simulink model "MPCisnm"  (R2023a)
settings: Solver=ode4  StartTime=0.0  StopTime=tsim  FixedStep=baseRate  RelTol=1e-6  AbsTol=1e-6
values from neighbouring files (symbols this model uses):
  ALGORITHM = 6    [Run_Initializer.m]
  con0 = [n*N, 2*N, N, N, N]    [Run_Initializer.m]
  Gamma1_el = 0.12    [Run_Initializer.m]
  Gamma1_sh = 0.005    [Run_Initializer.m]
  Gamma1_wr = 0.025    [Run_Initializer.m]
  Gamma2_el = 5    [Run_Initializer.m]
  Gamma2_sh = 5    [Run_Initializer.m]
  Gamma2_wr = 5    [Run_Initializer.m]
  Gamma3_el = 10    [Run_Initializer.m]
  Gamma3_sh = 40    [Run_Initializer.m]
  Gamma3_wr = 40    [Run_Initializer.m]
  Gamma4_el = 0.039    [Run_Initializer.m]
  Gamma4_sh = 0.015    [Run_Initializer.m]
  Gamma4_wr = 0.029    [Run_Initializer.m]
  Gamma5_el = 800    [Run_Initializer.m]
  Gamma5_sh = 800    [Run_Initializer.m]
  Gamma5_wr = 800    [Run_Initializer.m]
  Gamma6_el = 0.000001    (= 1e-06)    [Run_Initializer.m]
  Gamma6_sh = 0.005    [Run_Initializer.m]
  Gamma6_wr = 0.02    [Run_Initializer.m]
  init_states_BLACK = [ct;thetat0].'    [Run_Initializer.m]
  init_states_BLUE = [pobj1;0].'    [Run_Initializer.m]
  init_states_RED = xi(1:3).'    [Run_Initializer.m]
  Kd_elarm = 0.8    [Run_Initializer.m]
  Kd_sharm = 1.0    (= 1)    [Run_Initializer.m]
  Kd_wrarm = 0.6    [Run_Initializer.m]
  Kp_elarm = 1.2    [Run_Initializer.m]
  Kp_sharm = 1.5    [Run_Initializer.m]
  Kp_wrarm = 2    [Run_Initializer.m]
  maxiterations = 10    [Run_Initializer.m]
  N = 15    [Run_Initializer.m]    (also in theFastMPCSolver2.m = length(z)/9)
  Phi = 2*H + kappa*P.'*d2*P    [theFastMPCSolver2.m]
  Td = 2    [Run_Initializer.m]
  thetat_dot = 2.5 * d2r    (= 0.0436332312999)    [Run_Initializer.m]
  tol = 0.00015    [Run_Initializer.m]
  Tz_lim_elarm = .1    (= 0.1)    [Run_Initializer.m]
  Tz_lim_sharm = .1    (= 0.1)    [Run_Initializer.m]
  Tz_lim_wrarm = .1    (= 0.1)    [Run_Initializer.m]
  vobj1 = [0.00;0.00]    [Run_Initializer.m]
  vtar = [-0.005;0.005]    [Run_Initializer.m]
undefined symbols (not defined in the file or in its folder): a1, a2, a3, Ad, b0, b1, b2, b3, baseRate, cdockdeltax, cdockoa, Cmat, DiscIntNeverNeededParam, drop_states_ARM, drop_states_BLACK, drop_states_BLUE, drop_states_RED, ecoa, F_Black_X_nominal, F_Black_Y_nominal, F_Blue_X_nominal, F_Blue_Y_nominal, F_red_X_nominal, F_red_Y_nominal, F_thrusters_BLACK, F_thrusters_BLUE, F_thrusters_RED, Fmat, gamma, H, IBLACK, IBLUE, IDIST, IEE, IPROX, IRED, Kd_tb, Kd_tblue, Kd_tr, Kd_xb, Kd_xblue, Kd_xr, Kd_yb, Kd_yblue, Kd_yr, KOZ_actual, Kp_tb, Kp_tblue, Kp_tr, Kp_xb, Kp_xblue, Kp_xr, Kp_yb, Kp_yblue, Kp_yr, mBLACK, mBLUE, mDIST, mEE, mPROX ... (+31)
libraries: nvidiaSharedBlocks x8, simulink x8, dspsigops x6, dspstat3 x5, MainLibrary x4
(part 3 of 10)

== system MPCisnm/Phase #3: Experiment/Change BLUE Behavior ==
  Action Port : ActionPort  ActionPortLabel=if(u1 == 3 | u2 == 1)
  Constant1 : Constant  Value=Phase3_SubPhase2_End  SampleTime=-1
  Constant2 : Constant  Value=Phase3_SubPhase3_End  SampleTime=-1
  Constant3 : Constant  Value=Phase3_SubPhase4_End  SampleTime=-1
  Constant4 : Constant  Value=Phase3_SubPhase1_End  SampleTime=-1
  Experiment Sub-Phases : If  NumInputs=5  IfExpression=u1 < u2  ElseIfExpressions=(u1 < u3 & u1 >= u2),(u1 < u4 & u1 >= u3), (u1 < u5 & u1 >= u4)  ShowElse=off
  Sub-Phase #1 : Subsystem  TreatAsAtomicUnit=on
  "Sub-Phase #2 " : Subsystem  TreatAsAtomicUnit=on
  "Sub-Phase #3 " : Subsystem  TreatAsAtomicUnit=on
  Sub-Phase #4 : Subsystem  TreatAsAtomicUnit=on
  Universal_Time : DataStoreRead  DataStoreName=Univ_Time  IndexOptions=Index vector (dialog)  Indices=1  OutputSizes=1
  wires:
  Constant3/1 -> Experiment Sub-Phases/5
  Experiment Sub-Phases/4 -> Sub-Phase #4/Action
  Universal_Time/1 -> Experiment Sub-Phases/1
  Experiment Sub-Phases/1 -> Sub-Phase #1/Action
  Constant2/1 -> Experiment Sub-Phases/4
  Constant4/1 -> Experiment Sub-Phases/2
  Constant1/1 -> Experiment Sub-Phases/3
  Experiment Sub-Phases/3 -> "Sub-Phase #3 "/Action
  Experiment Sub-Phases/2 -> "Sub-Phase #2 "/Action

== system MPCisnm/Phase #3: Experiment/Change RED Behavior ==
  note: For experiments, it is usually desirable to have various sub-phases. The sub-phases are defined in the initializer; note that in the template only three sub-phases are present, but more can be added.
  Action Port : ActionPort  ActionPortLabel=if(u1 == 1 | u2 == 1)
  Constant1 : Constant  Value=Phase3_SubPhase2_End  SampleTime=-1
  Constant2 : Constant  Value=Phase3_SubPhase3_End  SampleTime=-1
  Constant3 : Constant  Value=Phase3_SubPhase4_End  SampleTime=-1
  Constant4 : Constant  Value=Phase3_SubPhase1_End  SampleTime=-1
  Experiment Sub-Phases : If  NumInputs=5  IfExpression=u1 < u2  ElseIfExpressions=(u1 < u3 & u1 >= u2),(u1 < u4 & u1 >= u3), (u1 < u5 & u1 >= u4)  ShowElse=off
  Sub-Phase #1 : Subsystem  TreatAsAtomicUnit=on
  "Sub-Phase #2 " : Subsystem  TreatAsAtomicUnit=on
  "Sub-Phase #3 " : Subsystem  TreatAsAtomicUnit=on
  Sub-Phase #4 : Subsystem  TreatAsAtomicUnit=on
  Universal_Time : DataStoreRead  DataStoreName=Univ_Time  IndexOptions=Index vector (dialog)  Indices=1  OutputSizes=1
  wires:
  Experiment Sub-Phases/1 -> Sub-Phase #1/Action
  Experiment Sub-Phases/2 -> "Sub-Phase #2 "/Action
  Universal_Time/1 -> Experiment Sub-Phases/1
  Experiment Sub-Phases/3 -> "Sub-Phase #3 "/Action
  Constant4/1 -> Experiment Sub-Phases/2
  Constant1/1 -> Experiment Sub-Phases/3
  Constant2/1 -> Experiment Sub-Phases/4
  Constant3/1 -> Experiment Sub-Phases/5
  Experiment Sub-Phases/4 -> Sub-Phase #4/Action

== system MPCisnm/Phase #4: Return Home/Change BLACK Behavior ==
  note: Additional Blocks
  note: PD Control Law - BLACK
  note: Additional blocks are stored here.
  note: A simple PD control law is used here to command the platform to it's initial position, as defined in the initializer.
  Action Port : ActionPort  ActionPortLabel=if(u1 == 2 | u2 == 1)
  BLACK_Fx : DataStoreWrite  DataStoreName=BLACK_Fx  IndexOptions=Index vector (dialog)  Indices=1  OutputSizes=1
  BLACK_Fy : DataStoreWrite  DataStoreName=BLACK_Fy  IndexOptions=Index vector (dialog)  Indices=1  OutputSizes=1
  BLACK_Tz : DataStoreWrite  DataStoreName=BLACK_Tz  IndexOptions=Index vector (dialog)  Indices=1  OutputSizes=1
  Constant : Constant  Value=0
  Data Store Write3 : DataStoreWrite  DataStoreName=Float_State  IndexOptions=Index vector (dialog)  Indices=1  OutputSizes=1
  Puck State : Constant
  wires:
  Puck State/1 -> Data Store Write3/1
  Constant/1 -> BLACK_Fx/1, BLACK_Fy/1, BLACK_Tz/1

== system MPCisnm/Phase #4: Return Home/Change BLUE Behavior ==
  note: PD Control Law - BLUE
  note: Additional blocks are stored here.
  note: A simple PD control law is used here to command the platform to it's initial position, as defined in the initializer.
  note: Additional Blocks
  Action Port : ActionPort  ActionPortLabel=if(u1 == 3 | u2 == 1)
  BLUE_Fx : DataStoreWrite  DataStoreName=BLUE_Fx  IndexOptions=Index vector (dialog)  Indices=1  OutputSizes=1
  BLUE_Fy : DataStoreWrite  DataStoreName=BLUE_Fy  IndexOptions=Index vector (dialog)  Indices=1  OutputSizes=1
  BLUE_Tz : DataStoreWrite  DataStoreName=BLUE_Tz  IndexOptions=Index vector (dialog)  Indices=1  OutputSizes=1
  Constant : Constant  Value=0
  Data Store Write3 : DataStoreWrite  DataStoreName=Float_State  IndexOptions=Index vector (dialog)  Indices=1  OutputSizes=1
  Puck State : Constant
  wires:
  Puck State/1 -> Data Store Write3/1
  Constant/1 -> BLUE_Tz/1, BLUE_Fx/1, BLUE_Fy/1

== system MPCisnm/Phase #4: Return Home/Change RED Behavior ==
  note: PD Control Law - RED
  note: Additional Blocks
  note: Additional blocks are stored above. Note that to control attitude using the RW, simply replace RED_Tz with RED_Tz_RW.
  note: A simple PD control law is used here to command the platform to it's initial position, as defined in the initializer.
  note: ARM Control Law - RED
  Action Port : ActionPort  ActionPortLabel=if(u1 == 1 | u2 == 1)
  Constant{,1..3,5..7} (7 alike) : Constant  Value=0
  Constant4 : Constant  Commented=on  Value=platformSelection
  Data Store Write : DataStoreWrite  DataStoreName=MPC_State  IndexOptions=Index vector (dialog)  Indices=1  OutputSizes=1
  Data Store Write1 : DataStoreWrite  DataStoreName=RED_ARM_Control_Mode  IndexOptions=Index vector (dialog)  Indices=1  OutputSizes=1
  Data Store Write3 : DataStoreWrite  DataStoreName=Float_State  IndexOptions=Index vector (dialog)  Indices=1  OutputSizes=1
  If : If  Commented=on  IfExpression=u1 == 4 | u1 == 5 | u1 == 10 | u1 == 11  ShowElse=off
  Puck State : Constant
  RED+ARM : Subsystem  Commented=on  TreatAsAtomicUnit=on
  RED_Fx : DataStoreWrite  DataStoreName=RED_Fx  IndexOptions=Index vector (dialog)  Indices=1  OutputSizes=1
  RED_Fy : DataStoreWrite  DataStoreName=RED_Fy  IndexOptions=Index vector (dialog)  Indices=1  OutputSizes=1
  RED_Tz : DataStoreWrite  DataStoreName=RED_Tz  IndexOptions=Index vector (dialog)  Indices=1  OutputSizes=1
  RED_Tz_RW : DataStoreWrite  DataStoreName=RED_Tz_RW  IndexOptions=Index vector (dialog)  Indices=1  OutputSizes=1
  RED_Tz_RW1 : DataStoreWrite  DataStoreName=RED_Tz_RW  IndexOptions=Index vector (dialog)  Indices=1  OutputSizes=1
  wires:
  Constant2/1 -> RED_Tz_RW1/1
  Puck State/1 -> Data Store Write3/1
  Constant4/1 -> If/1
  If/1 -> RED+ARM/Action
  Constant1/1 -> RED_Fy/1
  Constant/1 -> RED_Fx/1
  Constant3/1 -> RED_Tz/1
  Constant5/1 -> RED_Tz_RW/1
  Constant6/1 -> Data Store Write1/1
  Constant7/1 -> Data Store Write/1

== system MPCisnm/Phase #5: Hold Home/Change BLACK Behavior ==
  note: Additional Blocks
  note: PD Control Law - BLACK
  note: Additional blocks are stored here.
  note: A simple PD control law is used here to command the platform to it's initial position, as defined in the initializer.
  Action Port : ActionPort  ActionPortLabel=if(u1 == 2 | u2 == 1)
  BLACK_Fx : DataStoreWrite  DataStoreName=BLACK_Fx  IndexOptions=Index vector (dialog)  Indices=1  OutputSizes=1
  BLACK_Fy : DataStoreWrite  DataStoreName=BLACK_Fy  IndexOptions=Index vector (dialog)  Indices=1  OutputSizes=1
  BLACK_Tz : DataStoreWrite  DataStoreName=BLACK_Tz  IndexOptions=Index vector (dialog)  Indices=1  OutputSizes=1
  Data Store Write3 : DataStoreWrite  DataStoreName=Float_State  IndexOptions=Index vector (dialog)  Indices=1  OutputSizes=1
  Puck State : Constant
  Puck State1 : Constant  Value=0
  Puck State2 : Constant  Value=0
  Puck State3 : Constant  Value=0
  wires:
  Puck State2/1 -> BLACK_Fy/1
  Puck State3/1 -> BLACK_Tz/1
  Puck State1/1 -> BLACK_Fx/1
  Puck State/1 -> Data Store Write3/1

== system MPCisnm/Phase #5: Hold Home/Change BLUE Behavior ==
  note: PD Control Law - BLUE
  note: Additional blocks are stored here.
  note: A simple PD control law is used here to command the platform to it's initial position, as defined in the initializer.
  note: Additional Blocks
  Action Port : ActionPort  ActionPortLabel=if(u1 == 3 | u2 == 1)
  BLUE_Fx : DataStoreWrite  DataStoreName=BLUE_Fx  IndexOptions=Index vector (dialog)  Indices=1  OutputSizes=1
  BLUE_Fy : DataStoreWrite  DataStoreName=BLUE_Fy  IndexOptions=Index vector (dialog)  Indices=1  OutputSizes=1
  BLUE_Tz : DataStoreWrite  DataStoreName=BLUE_Tz  IndexOptions=Index vector (dialog)  Indices=1  OutputSizes=1
  Data Store Write3 : DataStoreWrite  DataStoreName=Float_State  IndexOptions=Index vector (dialog)  Indices=1  OutputSizes=1
  Puck State : Constant
  Puck State1 : Constant  Value=0
  Puck State2 : Constant  Value=0
  Puck State3 : Constant  Value=0
  wires:
  Puck State/1 -> Data Store Write3/1
  Puck State1/1 -> BLUE_Fx/1
  Puck State3/1 -> BLUE_Tz/1
  Puck State2/1 -> BLUE_Fy/1

== system MPCisnm/Phase #5: Hold Home/Change RED Behavior ==
  note: PD Control Law - RED
  note: Additional Blocks
  note: Additional blocks are stored above. Note that to control attitude using the RW, simply replace RED_Tz with RED_Tz_RW.
  note: A simple PD control law is used here to command the platform to it's initial position, as defined in the initializer.
  note: ARM Control Law - RED
  Action Port : ActionPort  ActionPortLabel=if(u1 == 1 | u2 == 1)
  Constant{,1..3,5..7} (7 alike) : Constant  Value=0
  Constant4 : Constant  Commented=on  Value=platformSelection
  Data Store Write : DataStoreWrite  DataStoreName=MPC_State  IndexOptions=Index vector (dialog)  Indices=1  OutputSizes=1
  Data Store Write1 : DataStoreWrite  DataStoreName=RED_ARM_Control_Mode  IndexOptions=Index vector (dialog)  Indices=1  OutputSizes=1
  Data Store Write3 : DataStoreWrite  DataStoreName=Float_State  IndexOptions=Index vector (dialog)  Indices=1  OutputSizes=1
  If : If  Commented=on  IfExpression=u1 == 4 | u1 == 5 | u1 == 10 | u1 == 11  ShowElse=off
  Puck State : Constant
  RED+ARM : Subsystem  Commented=on  TreatAsAtomicUnit=on
  RED_Fx : DataStoreWrite  DataStoreName=RED_Fx  IndexOptions=Index vector (dialog)  Indices=1  OutputSizes=1
  RED_Fy : DataStoreWrite  DataStoreName=RED_Fy  IndexOptions=Index vector (dialog)  Indices=1  OutputSizes=1
  RED_Tz : DataStoreWrite  DataStoreName=RED_Tz  IndexOptions=Index vector (dialog)  Indices=1  OutputSizes=1
  RED_Tz_RW : DataStoreWrite  DataStoreName=RED_Tz_RW  IndexOptions=Index vector (dialog)  Indices=1  OutputSizes=1
  RED_Tz_RW1 : DataStoreWrite  DataStoreName=RED_Tz_RW  IndexOptions=Index vector (dialog)  Indices=1  OutputSizes=1
  wires:
  Constant2/1 -> RED_Tz_RW1/1
  Puck State/1 -> Data Store Write3/1
  Constant4/1 -> If/1
  If/1 -> RED+ARM/Action
  Constant1/1 -> RED_Fy/1
  Constant/1 -> RED_Fx/1
  Constant3/1 -> RED_Tz/1
  Constant5/1 -> RED_Tz_RW/1
  Constant6/1 -> Data Store Write1/1
  Constant7/1 -> Data Store Write/1

== system MPCisnm/Phase #6: Clean Shutdown/Change BLACK Behavior ==
  note: At the end of the experiment, the pucks must be turned off.
  note: At the end of the experiment, all thrust and arms movement must cease.
  Action Port : ActionPort  ActionPortLabel=if(u1 == 2 | u2 == 1)
  BLACK_Fx : DataStoreWrite  DataStoreName=BLACK_Fx  IndexOptions=Index vector (dialog)  Indices=1  OutputSizes=1
  BLACK_Fy : DataStoreWrite  DataStoreName=BLACK_Fy  IndexOptions=Index vector (dialog)  Indices=1  OutputSizes=1
  BLACK_Tz : DataStoreWrite  DataStoreName=BLACK_Tz  IndexOptions=Index vector (dialog)  Indices=1  OutputSizes=1
  Constant3 : Constant  Value=0
  Constant4 : Constant  Value=0
  Constant5 : Constant  Value=0
  Data Store Write3 : DataStoreWrite  DataStoreName=Float_State  IndexOptions=Index vector (dialog)  Indices=1  OutputSizes=1
  Puck State : Constant  Value=0
  wires:
  Constant3/1 -> BLACK_Fx/1
  Constant5/1 -> BLACK_Tz/1
  Constant4/1 -> BLACK_Fy/1
  Puck State/1 -> Data Store Write3/1

== system MPCisnm/Phase #6: Clean Shutdown/Change BLUE Behavior ==
  note: Before getting good data, the platforms must NOT be floating. So, float is set to be "off".
  note: For the initialization phase, we do not want any thrust. Thus, all commanded forces are zero.
  Action Port : ActionPort  ActionPortLabel=if(u1 == 3 | u2 == 1)
  BLUE_Fx : DataStoreWrite  DataStoreName=BLUE_Fx  IndexOptions=Index vector (dialog)  Indices=1  OutputSizes=1
  BLUE_Fy : DataStoreWrite  DataStoreName=BLUE_Fy  IndexOptions=Index vector (dialog)  Indices=1  OutputSizes=1
  BLUE_Tz : DataStoreWrite  DataStoreName=BLUE_Tz  IndexOptions=Index vector (dialog)  Indices=1  OutputSizes=1
  Constant3 : Constant  Value=0
  Constant4 : Constant  Value=0
  Constant5 : Constant  Value=0
  Data Store Write4 : DataStoreWrite  DataStoreName=Float_State  IndexOptions=Index vector (dialog)  Indices=1  OutputSizes=1
  Puck State : Constant  Value=0
  wires:
  Constant3/1 -> BLUE_Fx/1
  Constant5/1 -> BLUE_Tz/1
  Constant4/1 -> BLUE_Fy/1
  Puck State/1 -> Data Store Write4/1

== system MPCisnm/Phase #6: Clean Shutdown/Change RED Behavior ==
  note: At the end of the experiment, the pucks must be turned off.
  note: At the end of the experiment, all thrust and arms movement must cease.
  note: Once the platform has settled, the RW must be slowly desaturated (assuming it has been used).
  Action Port : ActionPort  ActionPortLabel=if(u1 == 1 | u2 == 1)
  Constant{,1..3,7} (5 alike) : Constant  Value=0
  Data Store Write : DataStoreWrite  DataStoreName=MPC_State  IndexOptions=Index vector (dialog)  Indices=1  OutputSizes=1
  Data Store Write1 : DataStoreWrite  DataStoreName=RED_ARM_Control_Mode  IndexOptions=Index vector (dialog)  Indices=1  OutputSizes=1
  Data Store Write3 : DataStoreWrite  DataStoreName=Float_State  IndexOptions=Index vector (dialog)  Indices=1  OutputSizes=1
  Gain : Gain  Gain=-1
  Puck State : Constant  Value=0
  RED_Fx : DataStoreWrite  DataStoreName=RED_Fx  IndexOptions=Index vector (dialog)  Indices=1  OutputSizes=1
  RED_Fy : DataStoreWrite  DataStoreName=RED_Fy  IndexOptions=Index vector (dialog)  Indices=1  OutputSizes=1
  RED_Tz : DataStoreWrite  DataStoreName=RED_Tz  IndexOptions=Index vector (dialog)  Indices=1  OutputSizes=1
  RED_Tz_RW : DataStoreWrite  DataStoreName=RED_Tz_RW  IndexOptions=Index vector (dialog)  Indices=1  OutputSizes=1
  RED_dRz_Speed : DataStoreRead  DataStoreName=RED_dRz_RW_Sat  IndexOptions=Index vector (dialog)  Indices=1  OutputSizes=1
  Saturation : Saturate  UpperLimit=0.005  LowerLimit=-0.005
  wires:
  Constant/1 -> RED_Fx/1
  RED_dRz_Speed/1 -> Gain/1
  Saturation/1 -> RED_Tz_RW/1
  Constant1/1 -> RED_Fy/1
  Gain/1 -> Saturation/1
  Constant2/1 -> RED_Tz/1
  Puck State/1 -> Data Store Write3/1
  Constant3/1 -> Data Store Write1/1
  Constant7/1 -> Data Store Write/1

== system MPCisnm/PhaseSpace Camera Code/Initialize Universal Time (Simulation) ==
  Action Port : ActionPort  ActionPortLabel=elseif(u1 == 1)
  Set Universal Time (If this is a simulation) : Clock
  Universal_Time : DataStoreWrite  DataStoreName=Univ_Time  IndexOptions=Index vector (dialog)  Indices=1  OutputSizes=1
  wires:
  Set Universal Time (If this is a simulation)/1 -> Universal_Time/1

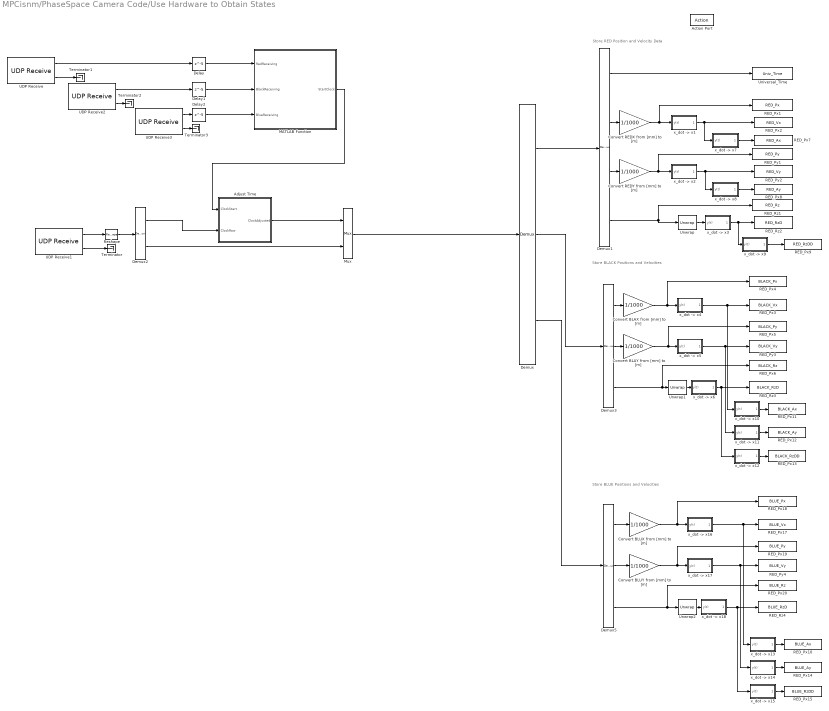
== system MPCisnm/PhaseSpace Camera Code/Use Hardware to Obtain States ==
  note: Store RED Position and Velocity Data
  note: Store BLUE Positions and Velocities
  note: Store BLACK Positions and Velocities
  Action Port : ActionPort  ActionPortLabel=if(u1 == 0)
  Adjust Time : Subsystem
  Convert BLAX from [mm] to [m] : Gain  Gain=1/1000
  Convert BLAY from [mm] to [m] : Gain  Gain=1/1000
  Convert BLUX from [mm] to [m] : Gain  Gain=1/1000
  Convert BLUY from [mm] to [m] : Gain  Gain=1/1000
  Convert REDX from [mm] to [m] : Gain  Gain=1/1000
  Convert REDY from [mm] to [m] : Gain  Gain=1/1000
  Delay : Delay  DelayLength=5
  Delay1 : Delay  DelayLength=5
  Delay2 : Delay  DelayLength=5
  Demux : Demux  Outputs=[4,3,3]
  Demux1 : Demux
  Demux2 : Demux  Outputs=[1,9]
  Demux3 : Demux  Outputs=3
  Demux5 : Demux  Outputs=3
  MATLAB Function : MATLAB Function  TreatAsAtomicUnit=on
  Mux : Mux  Inputs=2
  RED_Px1 : DataStoreWrite  DataStoreName=RED_Px  IndexOptions=Index vector (dialog)  Indices=1  OutputSizes=1
  RED_Px10 : DataStoreWrite  DataStoreName=BLUE_Ax  IndexOptions=Index vector (dialog)  Indices=1  OutputSizes=1
  RED_Px11 : DataStoreWrite  DataStoreName=BLACK_Ax  IndexOptions=Index vector (dialog)  Indices=1  OutputSizes=1
  RED_Px12 : DataStoreWrite  DataStoreName=BLACK_Ay  IndexOptions=Index vector (dialog)  Indices=1  OutputSizes=1
  RED_Px13 : DataStoreWrite  DataStoreName=BLACK_RzDD  IndexOptions=Index vector (dialog)  Indices=1  OutputSizes=1
  RED_Px14 : DataStoreWrite  DataStoreName=BLUE_Ay  IndexOptions=Index vector (dialog)  Indices=1  OutputSizes=1
  RED_Px15 : DataStoreWrite  DataStoreName=BLUE_RzDD  IndexOptions=Index vector (dialog)  Indices=1  OutputSizes=1
  RED_Px17 : DataStoreWrite  DataStoreName=BLUE_Vx  IndexOptions=Index vector (dialog)  Indices=1  OutputSizes=1
  RED_Px18 : DataStoreWrite  DataStoreName=BLUE_Px  IndexOptions=Index vector (dialog)  Indices=1  OutputSizes=1
  RED_Px19 : DataStoreWrite  DataStoreName=BLUE_Py  IndexOptions=Index vector (dialog)  Indices=1  OutputSizes=1
  RED_Px2 : DataStoreWrite  DataStoreName=RED_Vx  IndexOptions=Index vector (dialog)  Indices=1  OutputSizes=1
  RED_Px20 : DataStoreWrite  DataStoreName=BLUE_Rz  IndexOptions=Index vector (dialog)  Indices=1  OutputSizes=1
  RED_Px3 : DataStoreWrite  DataStoreName=BLACK_Vx  IndexOptions=Index vector (dialog)  Indices=1  OutputSizes=1
  RED_Px4 : DataStoreWrite  DataStoreName=BLACK_Px  IndexOptions=Index vector (dialog)  Indices=1  OutputSizes=1
  RED_Px5 : DataStoreWrite  DataStoreName=BLACK_Py  IndexOptions=Index vector (dialog)  Indices=1  OutputSizes=1
  RED_Px6 : DataStoreWrite  DataStoreName=BLACK_Rz  IndexOptions=Index vector (dialog)  Indices=1  OutputSizes=1
  RED_Px7 : DataStoreWrite  DataStoreName=RED_Ax  IndexOptions=Index vector (dialog)  Indices=1  OutputSizes=1
  RED_Px8 : DataStoreWrite  DataStoreName=RED_Ay  IndexOptions=Index vector (dialog)  Indices=1  OutputSizes=1
  RED_Px9 : DataStoreWrite  DataStoreName=RED_RzDD  IndexOptions=Index vector (dialog)  Indices=1  OutputSizes=1
  RED_Py1 : DataStoreWrite  DataStoreName=RED_Py  IndexOptions=Index vector (dialog)  Indices=1  OutputSizes=1
  RED_Py2 : DataStoreWrite  DataStoreName=RED_Vy  IndexOptions=Index vector (dialog)  Indices=1  OutputSizes=1
  RED_Py3 : DataStoreWrite  DataStoreName=BLACK_Vy  IndexOptions=Index vector (dialog)  Indices=1  OutputSizes=1
  RED_Py4 : DataStoreWrite  DataStoreName=BLUE_Vy  IndexOptions=Index vector (dialog)  Indices=1  OutputSizes=1
  RED_Rz1 : DataStoreWrite  DataStoreName=RED_Rz  IndexOptions=Index vector (dialog)  Indices=1  OutputSizes=1
  RED_Rz2 : DataStoreWrite  DataStoreName=RED_RzD  IndexOptions=Index vector (dialog)  Indices=1  OutputSizes=1
  RED_Rz3 : DataStoreWrite  DataStoreName=BLACK_RzD  IndexOptions=Index vector (dialog)  Indices=1  OutputSizes=1
  RED_Rz4 : DataStoreWrite  DataStoreName=BLUE_RzD  IndexOptions=Index vector (dialog)  Indices=1  OutputSizes=1
  Reshape : Reshape  OutputDimensionality=Customize  OutputDimensions=[10,1]
  Terminator{,1..3} (4 alike) : Terminator
  UDP Receive : nvidiaSharedBlocks/UDP Receive  localURL='0.0.0.0'  localPort=33001  remoteURL='0.0.0.0'  remotePort=-1  recvBufferSize=8192  signalDatatype=int32  dims=1  isVarSize=off  showBlockingTime=off  blockingTime=0  sampletime=-1  blockPlatform=NVIDIA
      settings: LibrarySourceBlock=nvidiaNetworklib/UDP Receive
  UDP Receive1 : nvidiaSharedBlocks/UDP Receive  localURL='0.0.0.0'  localPort=31534  remoteURL='0.0.0.0'  remotePort=-1  recvBufferSize=8192  signalDatatype=double  dims=10  isVarSize=off  showBlockingTime=off  blockingTime=0  sampletime=-1  blockPlatform=NVIDIA
  UDP Receive2 : nvidiaSharedBlocks/UDP Receive  localURL='0.0.0.0'  localPort=33002  remoteURL='0.0.0.0'  remotePort=-1  recvBufferSize=8192  signalDatatype=int32  dims=1  isVarSize=off  showBlockingTime=off  blockingTime=0  sampletime=-1  blockPlatform=NVIDIA
      settings: LibrarySourceBlock=nvidiaNetworklib/UDP Receive
  UDP Receive3 : nvidiaSharedBlocks/UDP Receive  localURL='0.0.0.0'  localPort=33003  remoteURL='0.0.0.0'  remotePort=-1  recvBufferSize=8192  signalDatatype=int32  dims=1  isVarSize=off  showBlockingTime=off  blockingTime=0  sampletime=-1  blockPlatform=NVIDIA
      settings: LibrarySourceBlock=nvidiaNetworklib/UDP Receive
  Universal_Time : DataStoreWrite  DataStoreName=Univ_Time  IndexOptions=Index vector (dialog)  Indices=1  OutputSizes=1
  Unwrap : dspsigops/Unwrap  tol=pi  InputProcessing=Columns as channels (frame based)  running=off
  Unwrap1 : dspsigops/Unwrap  tol=pi  InputProcessing=Columns as channels (frame based)  running=off
  Unwrap2 : dspsigops/Unwrap  tol=pi  InputProcessing=Columns as channels (frame based)  running=off
  "x_dot -> x1" : Subsystem
  "x_dot -> x10" : Subsystem
  "x_dot -> x11" : Subsystem
  "x_dot -> x12" : Subsystem
  "x_dot -> x13" : Subsystem
  "x_dot -> x14" : Subsystem
  "x_dot -> x15" : Subsystem
  "x_dot -> x16" : Subsystem
  "x_dot -> x17" : Subsystem
  "x_dot -> x18" : Subsystem
  "x_dot -> x2" : Subsystem
  "x_dot -> x3" : Subsystem
  "x_dot -> x4" : Subsystem
  "x_dot -> x5" : Subsystem
  "x_dot -> x6" : Subsystem
  "x_dot -> x7" : Subsystem
  "x_dot -> x8" : Subsystem
  "x_dot -> x9" : Subsystem
  wires:
  "x_dot -> x12"/1(dy(t)/dt) -> RED_Px13/1
  "x_dot -> x6"/1(dy(t)/dt) -> RED_Rz3/1, "x_dot -> x12"/1(y(t))
  Unwrap2/1 -> "x_dot -> x18"/1(y(t))
  Demux1/4 -> Unwrap/1, RED_Rz1/1
  Demux3/3 -> Unwrap1/1, RED_Px6/1
  Demux3/2 -> Convert BLAY from [mm] to [m]/1
  Demux5/2 -> Convert BLUY from [mm] to [m]/1
  "x_dot -> x1"/1(dy(t)/dt) -> "x_dot -> x7"/1(y(t)), RED_Px2/1
  Demux5/3 -> Unwrap2/1, RED_Px20/1
  Demux5/1 -> Convert BLUX from [mm] to [m]/1
  "x_dot -> x2"/1(dy(t)/dt) -> "x_dot -> x8"/1(y(t)), RED_Py2/1
  Demux1/3 -> Convert REDY from [mm] to [m]/1
  Demux/1 -> Demux1/1
  "x_dot -> x8"/1(dy(t)/dt) -> RED_Px8/1
  Unwrap/1 -> "x_dot -> x3"/1(y(t))
  Demux/2 -> Demux3/1
  "x_dot -> x10"/1(dy(t)/dt) -> RED_Px11/1
  "x_dot -> x3"/1(dy(t)/dt) -> "x_dot -> x9"/1(y(t)), RED_Rz2/1
  "x_dot -> x7"/1(dy(t)/dt) -> RED_Px7/1
  "x_dot -> x11"/1(dy(t)/dt) -> RED_Px12/1
  "x_dot -> x5"/1(dy(t)/dt) -> RED_Py3/1, "x_dot -> x11"/1(y(t))
  Unwrap1/1 -> "x_dot -> x6"/1(y(t))
  "x_dot -> x4"/1(dy(t)/dt) -> "x_dot -> x10"/1(y(t)), RED_Px3/1
  Demux3/1 -> Convert BLAX from [mm] to [m]/1
  Demux1/2 -> Convert REDX from [mm] to [m]/1
  "x_dot -> x9"/1(dy(t)/dt) -> RED_Px9/1
  UDP Receive1/1 -> Reshape/1
  UDP Receive1/2 -> Terminator/1
  Mux/1 -> Demux/1
  Demux/3 -> Demux5/1
  Convert REDX from [mm] to [m]/1 -> "x_dot -> x1"/1(y(t)), RED_Px1/1
  Convert REDY from [mm] to [m]/1 -> "x_dot -> x2"/1(y(t)), RED_Py1/1
  Convert BLAX from [mm] to [m]/1 -> "x_dot -> x4"/1(y(t)), RED_Px4/1
  Convert BLAY from [mm] to [m]/1 -> "x_dot -> x5"/1(y(t)), RED_Px5/1
  "x_dot -> x17"/1(dy(t)/dt) -> "x_dot -> x14"/1(y(t)), RED_Py4/1
  "x_dot -> x16"/1(dy(t)/dt) -> "x_dot -> x13"/1(y(t)), RED_Px17/1
  "x_dot -> x14"/1(dy(t)/dt) -> RED_Px14/1
  "x_dot -> x15"/1(dy(t)/dt) -> RED_Px15/1
  "x_dot -> x13"/1(dy(t)/dt) -> RED_Px10/1
  "x_dot -> x18"/1(dy(t)/dt) -> "x_dot -> x15"/1(y(t)), RED_Rz4/1
  Convert BLUX from [mm] to [m]/1 -> "x_dot -> x16"/1(y(t)), RED_Px18/1
  Convert BLUY from [mm] to [m]/1 -> "x_dot -> x17"/1(y(t)), RED_Px19/1
  Demux1/1 -> Universal_Time/1
  Reshape/1 -> Demux2/1
  Demux2/2 -> Mux/2
  Adjust Time/1(ClockAdjusted) -> Mux/1
  Demux2/1 -> Adjust Time/2(ClockRaw)
  UDP Receive3/2 -> Terminator3/1
  UDP Receive2/2 -> Terminator2/1
  UDP Receive/1 -> Delay/1
  UDP Receive/2 -> Terminator1/1
  UDP Receive3/1 -> Delay2/1
  UDP Receive2/1 -> Delay1/1
  Delay/1 -> MATLAB Function/1(RedReceiving)
  Delay1/1 -> MATLAB Function/2(BlackReceiving)
  Delay2/1 -> MATLAB Function/3(BlueReceiving)
  MATLAB Function/1(StartClock) -> Adjust Time/1(ClockStart)

== system MPCisnm/Platform Identification/Subsystem ==
  Action Port : ActionPort  ActionPortLabel=if(u1 == 0)
  Data Store Write : DataStoreWrite  DataStoreName=WhoAmI  IndexOptions=Index vector (dialog)  Indices=1  OutputSizes=1
  WhoAmI : MainLibrary/WhoAmI  SampleTime=baseRate
      settings: SourceProductName=SPOT Custom Library
  wires:
  WhoAmI/1 -> Data Store Write/1

== system MPCisnm/Robotic Arm Code/Change RED Behavior ==
  Action Port : ActionPort  ActionPortLabel=if(u1 == 1 & u2 == 0)
  Arm Control Mode : DataStoreRead  DataStoreName=RED_ARM_Control_Mode  IndexOptions=Index vector (dialog)  Indices=1  OutputSizes=1
  "Control Dynamixel Actuators in either Position, Current, or Speed Control Modes" : MainLibrary/Dynamixel Functions/Control Dynamixel Actuators in  either Position, Current, or Speed  Control Modes  POSITION_P_GAIN=400  POSITION_I_GAIN=0  POSITION_D_GAIN=200  MAX_POSITION=3072  MIN_POSITION=1024  MOVE_TIME=0  CURRENT_LIMIT=850  SPEED_P_GAIN=400  SPEED_I_GAIN=100  VELOCITY_LIMIT=50  ACCELERATION_TIME=0  SampleTime=baseRate
      settings: SourceProductName=SPOT Custom Library
  Elbow Command : DataStoreRead  DataStoreName=RED_Elbow_Command  IndexOptions=Index vector (dialog)  Indices=1  OutputSizes=1
  Shoulder Command : DataStoreRead  DataStoreName=RED_Shoulder_Command  IndexOptions=Index vector (dialog)  Indices=1  OutputSizes=1
  Wrist Command : DataStoreRead  DataStoreName=RED_Wrist_Command  IndexOptions=Index vector (dialog)  Indices=1  OutputSizes=1
  wires:
  Arm Control Mode/1 -> "Control Dynamixel Actuators in either Position, Current, or Speed Control Modes"/1
  Shoulder Command/1 -> "Control Dynamixel Actuators in either Position, Current, or Speed Control Modes"/2
  Elbow Command/1 -> "Control Dynamixel Actuators in either Position, Current, or Speed Control Modes"/3
  Wrist Command/1 -> "Control Dynamixel Actuators in either Position, Current, or Speed Control Modes"/4

== system MPCisnm/Send Data to TX2/Subsystem ==
  Action Port : ActionPort  ActionPortLabel=if(u1 == 0)
  BLACK_Px : DataStoreRead  DataStoreName=BLACK_Px  IndexOptions=Index vector (dialog)  Indices=1  OutputSizes=1
  BLACK_Py : DataStoreRead  DataStoreName=BLACK_Py  IndexOptions=Index vector (dialog)  Indices=1  OutputSizes=1
  BLACK_Rz : DataStoreRead  DataStoreName=BLACK_Rz  IndexOptions=Index vector (dialog)  Indices=1  OutputSizes=1
  BLACK_RzD : DataStoreRead  DataStoreName=BLACK_RzD  IndexOptions=Index vector (dialog)  Indices=1  OutputSizes=1
  BLACK_Vx : DataStoreRead  DataStoreName=BLACK_Vx  IndexOptions=Index vector (dialog)  Indices=1  OutputSizes=1
  BLACK_Vy : DataStoreRead  DataStoreName=BLACK_Vy  IndexOptions=Index vector (dialog)  Indices=1  OutputSizes=1
  BLUE_Px : DataStoreRead  DataStoreName=BLUE_Px  IndexOptions=Index vector (dialog)  Indices=1  OutputSizes=1
  BLUE_Py : DataStoreRead  DataStoreName=BLUE_Py  IndexOptions=Index vector (dialog)  Indices=1  OutputSizes=1
  BLUE_Rz : DataStoreRead  DataStoreName=BLUE_Rz  IndexOptions=Index vector (dialog)  Indices=1  OutputSizes=1
  BLUE_RzD : DataStoreRead  DataStoreName=BLUE_RzD  IndexOptions=Index vector (dialog)  Indices=1  OutputSizes=1
  BLUE_Vx : DataStoreRead  DataStoreName=BLUE_Vx  IndexOptions=Index vector (dialog)  Indices=1  OutputSizes=1
  BLUE_Vy : DataStoreRead  DataStoreName=BLUE_Vy  IndexOptions=Index vector (dialog)  Indices=1  OutputSizes=1
  Mux : Mux  Inputs=19
  RED_Px : DataStoreRead  DataStoreName=RED_Px  IndexOptions=Index vector (dialog)  Indices=1  OutputSizes=1
  "RED_Py " : DataStoreRead  DataStoreName=RED_Py  IndexOptions=Index vector (dialog)  Indices=1  OutputSizes=1
  RED_Rz : DataStoreRead  DataStoreName=RED_Rz  IndexOptions=Index vector (dialog)  Indices=1  OutputSizes=1
  "RED_Vx " : DataStoreRead  DataStoreName=RED_Vx  IndexOptions=Index vector (dialog)  Indices=1  OutputSizes=1
  RED_Vy : DataStoreRead  DataStoreName=RED_Vy  IndexOptions=Index vector (dialog)  Indices=1  OutputSizes=1
  RED_Vz : DataStoreRead  DataStoreName=RED_RzD  IndexOptions=Index vector (dialog)  Indices=1  OutputSizes=1
  Time : DataStoreRead  DataStoreName=Univ_Time  IndexOptions=Index vector (dialog)  Indices=1  OutputSizes=1
  UDP Send : nvidiaSharedBlocks/UDP Send  remoteURL='192.168.1.113'  remotePort=46875  localURL='0.0.0.0'  localPortSource=Automatically determine  localPort=-1  sampletime=-1  blockPlatform=NVIDIA  separateLengthPort=0
      settings: LibrarySourceBlock=nvidiaNetworklib/UDP Send
  wires:
  Mux/1 -> UDP Send/1
  BLUE_RzD/1 -> Mux/19
  Time/1 -> Mux/1
  RED_Px/1 -> Mux/2
  "RED_Py "/1 -> Mux/3
  RED_Rz/1 -> Mux/4
  "RED_Vx "/1 -> Mux/5
  RED_Vy/1 -> Mux/6
  RED_Vz/1 -> Mux/7
  BLACK_Px/1 -> Mux/8
  BLACK_Py/1 -> Mux/9
  BLACK_Rz/1 -> Mux/10
  BLACK_Vx/1 -> Mux/11
  BLACK_Vy/1 -> Mux/12
  BLACK_RzD/1 -> Mux/13
  BLUE_Px/1 -> Mux/14
  BLUE_Py/1 -> Mux/15
  BLUE_Rz/1 -> Mux/16
  BLUE_Vx/1 -> Mux/17
  BLUE_Vy/1 -> Mux/18

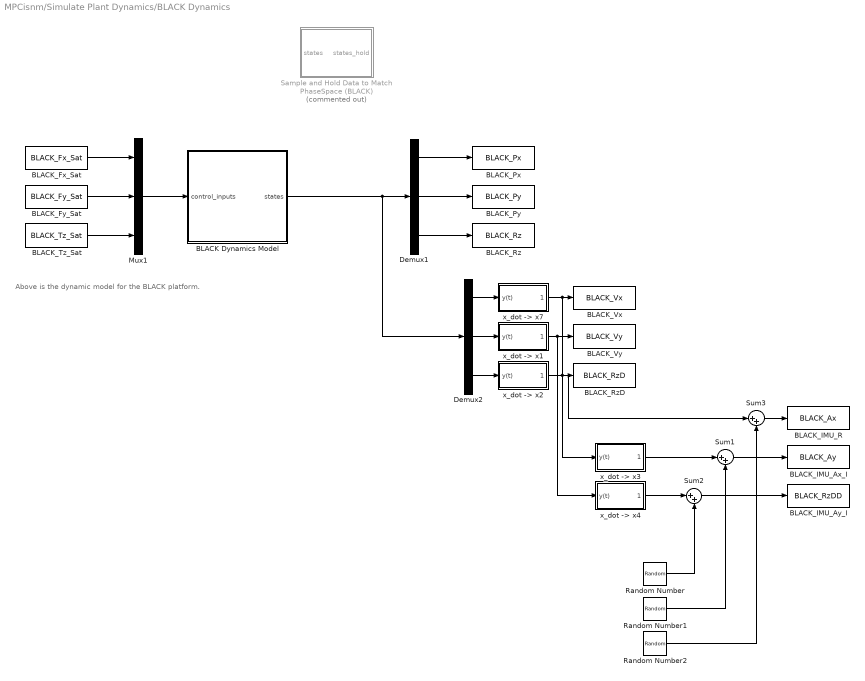
== system MPCisnm/Simulate Plant Dynamics/BLACK Dynamics ==
  note: Above is the dynamic model for the BLACK platform.
  BLACK Dynamics Model : Subsystem  SystemSampleTime=serverRate
  BLACK_Fx_Sat : DataStoreRead  DataStoreName=BLACK_Fx_Sat  IndexOptions=Index vector (dialog)  Indices=1  OutputSizes=1
  BLACK_Fy_Sat : DataStoreRead  DataStoreName=BLACK_Fy_Sat  IndexOptions=Index vector (dialog)  Indices=1  OutputSizes=1
  BLACK_IMU_Ax_I : DataStoreWrite  DataStoreName=BLACK_Ay  IndexOptions=Index vector (dialog)  Indices=1  OutputSizes=1
  BLACK_IMU_Ay_I : DataStoreWrite  DataStoreName=BLACK_RzDD  IndexOptions=Index vector (dialog)  Indices=1  OutputSizes=1
  BLACK_IMU_R : DataStoreWrite  DataStoreName=BLACK_Ax  IndexOptions=Index vector (dialog)  Indices=1  OutputSizes=1
  BLACK_Px : DataStoreWrite  DataStoreName=BLACK_Px  IndexOptions=Index vector (dialog)  Indices=1  OutputSizes=1
  BLACK_Py : DataStoreWrite  DataStoreName=BLACK_Py  IndexOptions=Index vector (dialog)  Indices=1  OutputSizes=1
  BLACK_Rz : DataStoreWrite  DataStoreName=BLACK_Rz  IndexOptions=Index vector (dialog)  Indices=1  OutputSizes=1
  BLACK_RzD : DataStoreWrite  DataStoreName=BLACK_RzD  IndexOptions=Index vector (dialog)  Indices=1  OutputSizes=1
  BLACK_Tz_Sat : DataStoreRead  DataStoreName=BLACK_Tz_Sat  IndexOptions=Index vector (dialog)  Indices=1  OutputSizes=1
  BLACK_Vx : DataStoreWrite  DataStoreName=BLACK_Vx  IndexOptions=Index vector (dialog)  Indices=1  OutputSizes=1
  BLACK_Vy : DataStoreWrite  DataStoreName=BLACK_Vy  IndexOptions=Index vector (dialog)  Indices=1  OutputSizes=1
  Demux1 : Demux  Outputs=3
  Demux2 : Demux  Outputs=3
  Mux1 : Mux  Inputs=3
  Random Number : RandomNumber  Variance=1.5e-6
  Random Number1 : RandomNumber  Variance=1.5e-6
  Random Number2 : RandomNumber  Variance=1.5e-6
  Sample and Hold Data to Match PhaseSpace (BLACK) : Subsystem  Commented=on
  Sum1 : Sum  Inputs=|++
  Sum2 : Sum  Inputs=|++
  Sum3 : Sum  Inputs=|++
  "x_dot -> x1" : Subsystem
  "x_dot -> x2" : Subsystem
  "x_dot -> x3" : Subsystem
  "x_dot -> x4" : Subsystem
  "x_dot -> x7" : Subsystem
  wires:
  BLACK_Fy_Sat/1 -> Mux1/2
  BLACK_Tz_Sat/1 -> Mux1/3
  Demux1/1 -> BLACK_Px/1
  "x_dot -> x7"/1(dy(t)/dt) -> "x_dot -> x3"/1(y(t)), BLACK_Vx/1
  "x_dot -> x2"/1(dy(t)/dt) -> Sum3/1, BLACK_RzD/1
  Demux1/2 -> BLACK_Py/1
  "x_dot -> x1"/1(dy(t)/dt) -> "x_dot -> x4"/1(y(t)), BLACK_Vy/1
  BLACK_Fx_Sat/1 -> Mux1/1
  Demux2/2 -> "x_dot -> x1"/1(y(t))
  Mux1/1 -> BLACK Dynamics Model/1(control_inputs)
  Demux2/3 -> "x_dot -> x2"/1(y(t))
  Demux1/3 -> BLACK_Rz/1
  Sum3/1 -> BLACK_IMU_R/1
  Demux2/1 -> "x_dot -> x7"/1(y(t))
  BLACK Dynamics Model/1(states) -> Demux2/1, Demux1/1
  Sum1/1 -> BLACK_IMU_Ax_I/1
  "x_dot -> x3"/1(dy(t)/dt) -> Sum1/1
  Sum2/1 -> BLACK_IMU_Ay_I/1
  Random Number/1 -> Sum2/2
  Random Number2/1 -> Sum3/2
  Random Number1/1 -> Sum1/2
  "x_dot -> x4"/1(dy(t)/dt) -> Sum2/1

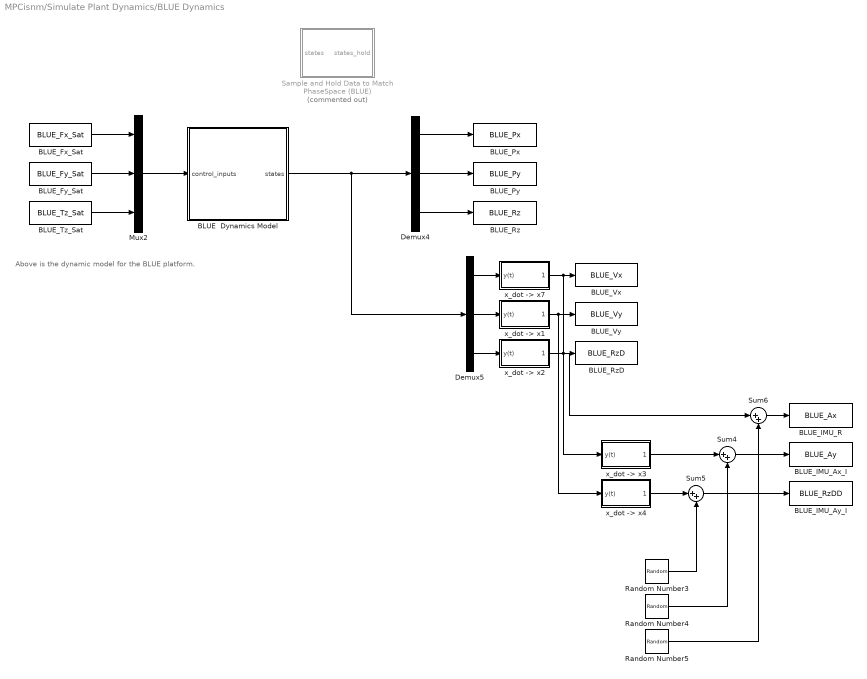
== system MPCisnm/Simulate Plant Dynamics/BLUE Dynamics ==
  note: Above is the dynamic model for the BLUE platform.
  BLUE  Dynamics Model : Subsystem  SystemSampleTime=serverRate
  "BLUE_Fx_Sat " : DataStoreRead  DataStoreName=BLUE_Fx_Sat  IndexOptions=Index vector (dialog)  Indices=1  OutputSizes=1
  BLUE_Fy_Sat : DataStoreRead  DataStoreName=BLUE_Fy_Sat  IndexOptions=Index vector (dialog)  Indices=1  OutputSizes=1
  BLUE_IMU_Ax_I : DataStoreWrite  DataStoreName=BLUE_Ay  IndexOptions=Index vector (dialog)  Indices=1  OutputSizes=1
  BLUE_IMU_Ay_I : DataStoreWrite  DataStoreName=BLUE_RzDD  IndexOptions=Index vector (dialog)  Indices=1  OutputSizes=1
  BLUE_IMU_R : DataStoreWrite  DataStoreName=BLUE_Ax  IndexOptions=Index vector (dialog)  Indices=1  OutputSizes=1
  "BLUE_Px " : DataStoreWrite  DataStoreName=BLUE_Px  IndexOptions=Index vector (dialog)  Indices=1  OutputSizes=1
  BLUE_Py : DataStoreWrite  DataStoreName=BLUE_Py  IndexOptions=Index vector (dialog)  Indices=1  OutputSizes=1
  BLUE_Rz : DataStoreWrite  DataStoreName=BLUE_Rz  IndexOptions=Index vector (dialog)  Indices=1  OutputSizes=1
  BLUE_RzD : DataStoreWrite  DataStoreName=BLUE_RzD  IndexOptions=Index vector (dialog)  Indices=1  OutputSizes=1
  BLUE_Tz_Sat : DataStoreRead  DataStoreName=BLUE_Tz_Sat  IndexOptions=Index vector (dialog)  Indices=1  OutputSizes=1
  BLUE_Vx : DataStoreWrite  DataStoreName=BLUE_Vx  IndexOptions=Index vector (dialog)  Indices=1  OutputSizes=1
  BLUE_Vy : DataStoreWrite  DataStoreName=BLUE_Vy  IndexOptions=Index vector (dialog)  Indices=1  OutputSizes=1
  Demux4 : Demux  Outputs=3
  Demux5 : Demux  Outputs=3
  Mux2 : Mux  Inputs=3
  Random Number3 : RandomNumber  Variance=1.5e-6
  Random Number4 : RandomNumber  Variance=1.5e-6
  Random Number5 : RandomNumber  Variance=1.5e-6
  Sample and Hold Data to Match PhaseSpace (BLUE) : Subsystem  Commented=on
  Sum4 : Sum  Inputs=|++
  Sum5 : Sum  Inputs=|++
  Sum6 : Sum  Inputs=|++
  "x_dot -> x1" : Subsystem
  "x_dot -> x2" : Subsystem
  "x_dot -> x3" : Subsystem
  "x_dot -> x4" : Subsystem
  "x_dot -> x7" : Subsystem
  wires:
  Demux5/3 -> "x_dot -> x2"/1(y(t))
  Demux4/1 -> "BLUE_Px "/1
  Demux4/2 -> BLUE_Py/1
  "BLUE_Fx_Sat "/1 -> Mux2/1
  BLUE_Fy_Sat/1 -> Mux2/2
  Demux5/1 -> "x_dot -> x7"/1(y(t))
  BLUE_Tz_Sat/1 -> Mux2/3
  Demux4/3 -> BLUE_Rz/1
  "x_dot -> x1"/1(dy(t)/dt) -> "x_dot -> x4"/1(y(t)), BLUE_Vy/1
  Mux2/1 -> BLUE  Dynamics Model/1(control_inputs)
  "x_dot -> x7"/1(dy(t)/dt) -> "x_dot -> x3"/1(y(t)), BLUE_Vx/1
  Sum5/1 -> BLUE_IMU_Ay_I/1
  "x_dot -> x2"/1(dy(t)/dt) -> Sum6/1, BLUE_RzD/1
  Sum4/1 -> BLUE_IMU_Ax_I/1
  Demux5/2 -> "x_dot -> x1"/1(y(t))
  Random Number3/1 -> Sum5/2
  "x_dot -> x3"/1(dy(t)/dt) -> Sum4/1
  "x_dot -> x4"/1(dy(t)/dt) -> Sum5/1
  Random Number4/1 -> Sum4/2
  Sum6/1 -> BLUE_IMU_R/1
  Random Number5/1 -> Sum6/2
  BLUE  Dynamics Model/1(states) -> Demux5/1, Demux4/1

== system MPCisnm/Simulate Plant Dynamics/RED and ARM Dynamics ==
  Constant : Constant  Value=platformSelection
  If : If  IfExpression=u1 == 4 | u1 == 5 | u1 == 10 | u1 == 11
  RED + ARM : Subsystem  TreatAsAtomicUnit=on
  RED Only : Subsystem  TreatAsAtomicUnit=on
  wires:
  If/1 -> RED + ARM/Action
  Constant/1 -> If/1
  If/2 -> RED Only/Action

== system MPCisnm/Subsystem/If Action Subsystem ==
  Action Port : ActionPort  ActionPortLabel=if(u1 == u2)
  Constant : Constant
  Data Store Read : DataStoreRead  DataStoreName=TRIGGER  IndexOptions=Index vector (dialog)  Indices=1  OutputSizes=1
  Data Store Write : DataStoreWrite  DataStoreName=COUNTER  IndexOptions=Index vector (dialog)  Indices=1  OutputSizes=1
  Data Store Write1 : DataStoreWrite  DataStoreName=TRIGGER  IndexOptions=Index vector (dialog)  Indices=1  OutputSizes=1
  If : If  IfExpression=u1 > 0.5
  If Action Subsystem : Subsystem  TreatAsAtomicUnit=on
  If Action Subsystem1 : Subsystem  TreatAsAtomicUnit=on
  Merge : Merge
  wires:
  Constant/1 -> Data Store Write/1
  Data Store Read/1 -> If/1
  If/1 -> If Action Subsystem/Action
  If/2 -> If Action Subsystem1/Action
  If Action Subsystem1/1(Out1) -> Merge/2
  If Action Subsystem/1(Out1) -> Merge/1
  Merge/1 -> Data Store Write1/1

== system MPCisnm/Subsystem/If Action Subsystem1 ==
  Action Port : ActionPort  ActionPortLabel=else
  Constant : Constant
  Data Store Read : DataStoreRead  DataStoreName=COUNTER  IndexOptions=Index vector (dialog)  Indices=1  OutputSizes=1
  Data Store Write : DataStoreWrite  DataStoreName=COUNTER  IndexOptions=Index vector (dialog)  Indices=1  OutputSizes=1
  Sum : Sum  Inputs=|++
  wires:
  Constant/1 -> Sum/2
  Data Store Read/1 -> Sum/1
  Sum/1 -> Data Store Write/1

== system MPCisnm/Subsystem/If Action Subsystem2 ==
  Action Port : ActionPort  ActionPortLabel=if(u1 > 0)
  Data Store Read : DataStoreRead  DataStoreName=TRIGGER  IndexOptions=Index vector (dialog)  Indices=1  OutputSizes=1
  Out1 : Outport
  wires:
  Data Store Read/1 -> Out1/1

== system MPCisnm/Subsystem/If Action Subsystem3 ==
  Action Port : ActionPort  ActionPortLabel=else
  Constant : Constant  Value=0
  Out1 : Outport
  wires:
  Constant/1 -> Out1/1

== system MPCisnm/Thruster Control Code/Change BLACK Behavior ==
  note: Calculate the percentage of time each thruster must be on, and send to the PWM blocks.
  note: Using the attitude, rotate the forces into the body frame.
  note: Calculate which thrusters must be turned on and for how long.
  Action Port : ActionPort  ActionPortLabel=if(u1 == 2 | u2 == 1)
  BLACK_Fx : DataStoreRead  DataStoreName=BLACK_Fx  IndexOptions=Index vector (dialog)  Indices=1  OutputSizes=1
  BLACK_Fy : DataStoreRead  DataStoreName=BLACK_Fy  IndexOptions=Index vector (dialog)  Indices=1  OutputSizes=1
  BLACK_Rz : DataStoreRead  DataStoreName=BLACK_Rz  IndexOptions=Index vector (dialog)  Indices=1  OutputSizes=1
  BLACK_Tz : DataStoreRead  DataStoreName=BLACK_Tz  IndexOptions=Index vector (dialog)  Indices=1  OutputSizes=1
  Calculate Thruster ON/OFF : Subsystem
  Mux : Mux  Inputs=2
  Mux1 : Mux  Inputs=2
  Rotate Forces to Body : Subsystem
  BLACK PWM : Outport  VectorParamsAs1DForOutWhenUnconnected=off
  wires:
  Rotate Forces to Body/1(F_b) -> Mux1/1
  Calculate Thruster ON/OFF/1(ThrusterPWM) -> BLACK PWM/1
  BLACK_Rz/1 -> Rotate Forces to Body/2(Rz)
  Mux/1 -> Rotate Forces to Body/1("F_I ")
  Mux1/1 -> Calculate Thruster ON/OFF/1("[Fx_b; Fy_b; Tz]")
  BLACK_Fx/1 -> Mux/1
  BLACK_Fy/1 -> Mux/2
  BLACK_Tz/1 -> Mux1/2

== system MPCisnm/Thruster Control Code/Change BLUE Behavior ==
  note: Calculate the percentage of time each thruster must be on, and send to the PWM blocks.
  note: Using the attitude, rotate the forces into the body frame.
  note: Calculate which thrusters must be turned on and for how long.
  Action Port : ActionPort  ActionPortLabel=if(u1 == 3 | u2 == 1)
  BLUE_Fx : DataStoreRead  DataStoreName=BLUE_Fx  IndexOptions=Index vector (dialog)  Indices=1  OutputSizes=1
  BLUE_Fy : DataStoreRead  DataStoreName=BLUE_Fy  IndexOptions=Index vector (dialog)  Indices=1  OutputSizes=1
  BLUE_Rz : DataStoreRead  DataStoreName=BLUE_Rz  IndexOptions=Index vector (dialog)  Indices=1  OutputSizes=1
  BLUE_Tz : DataStoreRead  DataStoreName=BLUE_Tz  IndexOptions=Index vector (dialog)  Indices=1  OutputSizes=1
  Calculate Thruster ON/OFF : Subsystem
  Mux : Mux  Inputs=2
  Mux1 : Mux  Inputs=2
  Rotate Forces to Body : Subsystem
  BLUE PWM : Outport  VectorParamsAs1DForOutWhenUnconnected=off
  wires:
  Rotate Forces to Body/1(F_b) -> Mux1/1
  Calculate Thruster ON/OFF/1(ThrusterPWM) -> BLUE PWM/1
  BLUE_Rz/1 -> Rotate Forces to Body/2(Rz)
  Mux/1 -> Rotate Forces to Body/1("F_I ")
  Mux1/1 -> Calculate Thruster ON/OFF/1("[Fx_b; Fy_b; Tz]")
  BLUE_Fx/1 -> Mux/1
  BLUE_Fy/1 -> Mux/2
  BLUE_Tz/1 -> Mux1/2

== system MPCisnm/Thruster Control Code/Change RED Behavior ==
  note: Calculate which thrusters must be turned on and for how long.
  note: Using the attitude, rotate the forces into the body frame.
  note: Calculate the percentage of time each thruster must be on, and send to the PWM blocks.
  Action Port : ActionPort  ActionPortLabel=if(u1 == 1 | u2 == 1)
  Calculate Thruster ON/OFF : Subsystem
  Mux : Mux  Inputs=2
  Mux1 : Mux  Inputs=2
  RED_Fx : DataStoreRead  DataStoreName=RED_Fx  IndexOptions=Index vector (dialog)  Indices=1  OutputSizes=1
  RED_Fy : DataStoreRead  DataStoreName=RED_Fy  IndexOptions=Index vector (dialog)  Indices=1  OutputSizes=1
  RED_Rz : DataStoreRead  DataStoreName=RED_Rz  IndexOptions=Index vector (dialog)  Indices=1  OutputSizes=1
  RED_Tz : DataStoreRead  DataStoreName=RED_Tz  IndexOptions=Index vector (dialog)  Indices=1  OutputSizes=1
  Rotate Forces to Body : Subsystem
  RED PWM : Outport  VectorParamsAs1DForOutWhenUnconnected=off
  wires:
  Mux/1 -> Rotate Forces to Body/1("F_I ")
  Mux1/1 -> Calculate Thruster ON/OFF/1("[Fx_b; Fy_b; Tz]")
  RED_Rz/1 -> Rotate Forces to Body/2(Rz)
  Rotate Forces to Body/1(F_b) -> Mux1/1
  Calculate Thruster ON/OFF/1(ThrusterPWM) -> RED PWM/1
  RED_Fx/1 -> Mux/1
  RED_Fy/1 -> Mux/2
  RED_Tz/1 -> Mux1/2

== system MPCisnm/Phase #2: Initial Position/Change BLACK Behavior/Custom Discrete PD (Attitude) ==
  ez : Inport
  Sum3 : Sum
  kd_tb : Gain  Gain=Kd_tb
  kp_tb : Gain  Gain=Kp_tb
  "x_dot -> x1" : Subsystem
  Tz : Outport  VectorParamsAs1DForOutWhenUnconnected=off
  wires:
  kd_tb/1 -> Sum3/1
  Sum3/1 -> Tz/1
  kp_tb/1 -> Sum3/2
  "x_dot -> x1"/1(dy(t)/dt) -> kd_tb/1
  ez/1 -> "x_dot -> x1"/1(y(t)), kp_tb/1

== system MPCisnm/Phase #2: Initial Position/Change BLACK Behavior/Custom Discrete PD (X-Position) ==
  ex : Inport
  Sum3 : Sum
  kd_xb : Gain  Gain=Kd_xb
  kp_xb : Gain  Gain=Kp_xb
  "x_dot -> x1" : Subsystem
  Fx : Outport  VectorParamsAs1DForOutWhenUnconnected=off
  wires:
  kd_xb/1 -> Sum3/1
  ex/1 -> "x_dot -> x1"/1(y(t)), kp_xb/1
  kp_xb/1 -> Sum3/2
  "x_dot -> x1"/1(dy(t)/dt) -> kd_xb/1
  Sum3/1 -> Fx/1

== system MPCisnm/Phase #2: Initial Position/Change BLACK Behavior/Custom Discrete PD (Y-Position) ==
  ey : Inport
  Sum3 : Sum
  kd_yb : Gain  Gain=Kd_yb
  kp_yb : Gain  Gain=Kp_yb
  "x_dot -> x1" : Subsystem
  Fy : Outport  VectorParamsAs1DForOutWhenUnconnected=off
  wires:
  kd_yb/1 -> Sum3/1
  Sum3/1 -> Fy/1
  kp_yb/1 -> Sum3/2
  "x_dot -> x1"/1(dy(t)/dt) -> kd_yb/1
  ey/1 -> "x_dot -> x1"/1(y(t)), kp_yb/1

== system MPCisnm/Phase #2: Initial Position/Change BLACK Behavior/Hough Control ==
  Ref : Inport
  Act : Inport  Port=2
  MATLAB Function2 : MATLAB Function  TreatAsAtomicUnit=on
  MATLAB Function3 : MATLAB Function  TreatAsAtomicUnit=on
  MATLAB Function4 : MATLAB Function  TreatAsAtomicUnit=on
  Subtract2 : Sum  Inputs=+-
  Err : Outport  VectorParamsAs1DForOutWhenUnconnected=off
  wires:
  MATLAB Function4/1(e_out) -> Err/1
  MATLAB Function2/1(Oy) -> MATLAB Function4/1(Oy)
  Subtract2/1 -> MATLAB Function4/2(e_in)
  MATLAB Function2/2(Ox) -> Subtract2/1
  Act/1 -> MATLAB Function3/1(z)
  Ref/1 -> MATLAB Function2/1(z)
  MATLAB Function3/1(Ox) -> Subtract2/2

== system MPCisnm/Phase #2: Initial Position/Change BLUE Behavior/Custom Discrete PD (Attitude) ==
  ez : Inport
  Sum3 : Sum
  kd_tb : Gain  Gain=Kd_tblue
  kp_tb : Gain  Gain=Kp_tblue
  "x_dot -> x1" : Subsystem
  Tz : Outport  VectorParamsAs1DForOutWhenUnconnected=off
  wires:
  kd_tb/1 -> Sum3/1
  Sum3/1 -> Tz/1
  kp_tb/1 -> Sum3/2
  "x_dot -> x1"/1(dy(t)/dt) -> kd_tb/1
  ez/1 -> "x_dot -> x1"/1(y(t)), kp_tb/1

== system MPCisnm/Phase #2: Initial Position/Change BLUE Behavior/Custom Discrete PD (X-Position) ==
  ex : Inport
  Sum3 : Sum
  kd_xb : Gain  Gain=Kd_xblue
  kp_xb : Gain  Gain=Kp_xblue
  "x_dot -> x1" : Subsystem
  Fx : Outport  VectorParamsAs1DForOutWhenUnconnected=off
  wires:
  kd_xb/1 -> Sum3/1
  ex/1 -> "x_dot -> x1"/1(y(t)), kp_xb/1
  kp_xb/1 -> Sum3/2
  "x_dot -> x1"/1(dy(t)/dt) -> kd_xb/1
  Sum3/1 -> Fx/1

== system MPCisnm/Phase #2: Initial Position/Change BLUE Behavior/Custom Discrete PD (Y-Position) ==
  ey : Inport
  Sum3 : Sum
  kd_yb : Gain  Gain=Kd_yblue
  kp_yb : Gain  Gain=Kp_yblue
  "x_dot -> x1" : Subsystem
  Fy : Outport  VectorParamsAs1DForOutWhenUnconnected=off
  wires:
  kd_yb/1 -> Sum3/1
  Sum3/1 -> Fy/1
  kp_yb/1 -> Sum3/2
  "x_dot -> x1"/1(dy(t)/dt) -> kd_yb/1
  ey/1 -> "x_dot -> x1"/1(y(t)), kp_yb/1

== system MPCisnm/Phase #2: Initial Position/Change BLUE Behavior/Hough Control ==
  Ref : Inport
  Act : Inport  Port=2
  MATLAB Function2 : MATLAB Function  TreatAsAtomicUnit=on
  MATLAB Function3 : MATLAB Function  TreatAsAtomicUnit=on
  MATLAB Function4 : MATLAB Function  TreatAsAtomicUnit=on
  Subtract2 : Sum  Inputs=+-
  Err : Outport  VectorParamsAs1DForOutWhenUnconnected=off
  wires:
  MATLAB Function4/1(e_out) -> Err/1
  MATLAB Function2/1(Oy) -> MATLAB Function4/1(Oy)
  Subtract2/1 -> MATLAB Function4/2(e_in)
  MATLAB Function2/2(Ox) -> Subtract2/1
  Act/1 -> MATLAB Function3/1(z)
  Ref/1 -> MATLAB Function2/1(z)
  MATLAB Function3/1(Ox) -> Subtract2/2

== system MPCisnm/Phase #2: Initial Position/Change RED Behavior/Custom Discrete PD (Attitude) ==
  ez : Inport
  Sum3 : Sum
  kd_tr : Gain  Gain=Kd_tr
  kp_tr : Gain  Gain=Kp_tr
  "x_dot -> x2" : Subsystem
  Tz : Outport  VectorParamsAs1DForOutWhenUnconnected=off
  wires:
  kd_tr/1 -> Sum3/1
  Sum3/1 -> Tz/1
  kp_tr/1 -> Sum3/2
  "x_dot -> x2"/1(dy(t)/dt) -> kd_tr/1
  ez/1 -> "x_dot -> x2"/1(y(t)), kp_tr/1

== system MPCisnm/Phase #2: Initial Position/Change RED Behavior/Custom Discrete PD (X-Position) ==
  ex : Inport
  Sum3 : Sum
  kd_xr : Gain  Gain=Kd_xr
  kp_xr : Gain  Gain=Kp_xr
  "x_dot -> x2" : Subsystem
  Fx : Outport  VectorParamsAs1DForOutWhenUnconnected=off
  wires:
  kd_xr/1 -> Sum3/1
  ex/1 -> "x_dot -> x2"/1(y(t)), kp_xr/1
  kp_xr/1 -> Sum3/2
  "x_dot -> x2"/1(dy(t)/dt) -> kd_xr/1
  Sum3/1 -> Fx/1

== system MPCisnm/Phase #2: Initial Position/Change RED Behavior/Custom Discrete PD (Y-Position) ==
  ey : Inport
  Sum3 : Sum
  kd_yr : Gain  Gain=Kd_yr
  kp_yr : Gain  Gain=Kp_yr
  "x_dot -> x2" : Subsystem
  Fy : Outport  VectorParamsAs1DForOutWhenUnconnected=off
  wires:
  kd_yr/1 -> Sum3/1
  Sum3/1 -> Fy/1
  kp_yr/1 -> Sum3/2
  "x_dot -> x2"/1(dy(t)/dt) -> kd_yr/1
  ey/1 -> "x_dot -> x2"/1(y(t)), kp_yr/1

== system MPCisnm/Phase #2: Initial Position/Change RED Behavior/Hough Control ==
  Ref : Inport
  Act : Inport  Port=2
  MATLAB Function2 : MATLAB Function  TreatAsAtomicUnit=on
  MATLAB Function3 : MATLAB Function  TreatAsAtomicUnit=on
  MATLAB Function4 : MATLAB Function  TreatAsAtomicUnit=on
  Subtract2 : Sum  Inputs=+-
  Err : Outport  VectorParamsAs1DForOutWhenUnconnected=off
  wires:
  MATLAB Function4/1(e_out) -> Err/1
  MATLAB Function2/1(Oy) -> MATLAB Function4/1(Oy)
  Subtract2/1 -> MATLAB Function4/2(e_in)
  MATLAB Function2/2(Ox) -> Subtract2/1
  Act/1 -> MATLAB Function3/1(z)
  Ref/1 -> MATLAB Function2/1(z)
  MATLAB Function3/1(Ox) -> Subtract2/2
